simulink model "untitled"  (R2020a)
settings: Solver=FixedStepAuto  StartTime=0.0  StopTime=10.0  FixedStep=0.00001  RelTol=1e-3
undefined symbols (not defined in the file): fp, fref, L, R, T, vdc
libraries: simulink x1
settings Model: Creator=ABO-CHIFA  LastModifiedBy=ABO-CHIFA

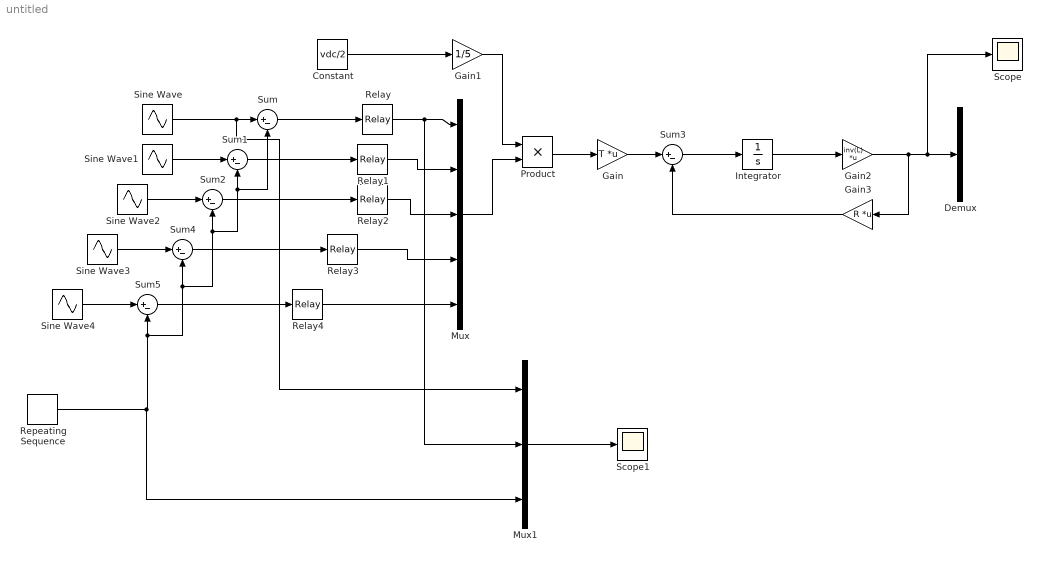
== system untitled ==
  Constant : Constant  Value=vdc/2
  Demux : Demux  Outputs=5
  Gain : Gain  Gain=T  Multiplication=Matrix(K*u)
  Gain1 : Gain  Gain=1/5
  Gain2 : Gain  Gain=inv(L)  Multiplication=Matrix(K*u)
  Gain3 : Gain  Gain=R  Multiplication=Matrix(K*u)
  Integrator : Integrator
  Mux : Mux  Inputs=5
  Mux1 : Mux  Inputs=3
  Product : Product
  Relay{,1..4} (5 alike) : Relay  OnSwitchValue=0.1  OffSwitchValue=-0.1  OffOutputValue=-1
  Repeating Sequence : simulink/Sources/Repeating Sequence  rep_seq_t=[0 1/(4*fp) 1/(3*fp) 1/(2*fp) 1/fp]  rep_seq_y=[-1 1 -1 1 -1]
  Scope : Scope
  Scope1 : Scope
  Sine Wave : Sin  Amplitude=0.8  Frequency=2*pi*fref  SampleTime=0
  Sine Wave1 : Sin  Amplitude=0.8  Frequency=2*pi*fref  Phase=2*pi/5  SampleTime=0
  Sine Wave2 : Sin  Amplitude=0.8  Frequency=2*pi*fref  Phase=4*pi/5  SampleTime=0
  Sine Wave3 : Sin  Amplitude=0.8  Frequency=2*pi*fref  Phase=6*pi/5  SampleTime=0
  Sine Wave4 : Sin  Amplitude=0.8  Frequency=2*pi*fref  Phase=8*pi/5  SampleTime=0
  Sum{,1..5} (6 alike) : Sum  Inputs=|+-
  wires:
  Mux/1 -> Product/2
  Product/1 -> Gain/1
  Gain1/1 -> Product/1
  Constant/1 -> Gain1/1
  Relay/1 -> Mux1/2, Mux/1
  Relay1/1 -> Mux/2
  Relay2/1 -> Mux/3
  Sum/1 -> Relay/1
  Sum1/1 -> Relay1/1
  Sine Wave/1 -> Mux1/1, Sum/1
  Sine Wave1/1 -> Sum1/1
  Sum2/1 -> Relay2/1
  Sine Wave2/1 -> Sum2/1
  Sine Wave3/1 -> Sum4/1
  Sine Wave4/1 -> Sum5/1
  Repeating Sequence/1 -> Mux1/3, Sum/2, Sum1/2, Sum2/2, Sum4/2, Sum5/2
  Relay3/1 -> Mux/4
  Sum4/1 -> Relay3/1
  Relay4/1 -> Mux/5
  Sum5/1 -> Relay4/1
  Gain/1 -> Sum3/1
  Sum3/1 -> Integrator/1
  Integrator/1 -> Gain2/1
  Gain3/1 -> Sum3/2
  Gain2/1 -> Gain3/1, Scope/1, Demux/1
  Mux1/1 -> Scope1/1
